simulink model "joint_impedance_control"  (R2019a)
settings: Solver=FixedStepDiscrete  StartTime=0.0  StopTime=inf  FixedStep=0.001  RelTol=1e-3
PreLoadFcn:
  | set_param(gcs, 'RTWSystemTargetFile', 'franka_emika_panda.tlc');
  | 
  | demos_common_configs();
  | collision_behavior = ones(1,52)*100;
libraries: franka_simulink_library x6, simulink x1
settings Model: SimulationMode=external  ExtModeTrigDuration=10000  Creator=vasi_ko  LastModifiedBy=konstantinosvasios
settings DataIOCC: LimitDataPoints=on  SaveFormat=Array  ReturnWorkspaceOutputs=off
settings OptimizationCC: EnhancedBackFolding=on  OptimizeBlockOrder=speed  DifferentSizesBufferReuse=on  OptimizationCustomize=off
settings DebuggingCC: SolverPrmCheckMsg=warning  ParameterTunabilityLossMsg=error  SFUnexpectedBacktrackingDiag=warning  SFNoUnconditionalDefaultTransitionDiag=warning  SFExecutionAtInitializationDiag=none  ArithmeticOperatorsInVariantConditions=warning
settings HardwareCC: ProdBitPerLong=64  ProdHWDeviceType=Intel->x86-64 (Linux 64)
settings ModelReferenceCC: PropagateSignalLabelsOutOfModel=off
settings SFSimCC: SimUseLocalCustomCode=off  MATLABDynamicMemAlloc=off
settings RTWCC: Description=Generic Real-Time Target  SystemTargetFile=franka_emika_panda.tlc  RTWUseLocalCustomCode=off  Toolchain=Franka Simulink | gmake (64-bit linux)  BuildConfiguration=Faster Runs  TargetLang=C++
settings CodeAppCC: OperatorAnnotations=on
settings STFCustomTargetCC: TargetLangStandard=C99 (ISO)  ModelReferenceCompliant=off  MatFileLogging=on  UseToolchainInfoCompliant=on  SystemTargetFile=franka_emika_panda.tlc
settings GRTTargetCC: ModelReferenceCompliant=off  ParMdlRefBuildCompliant=off  CompOptLevelCompliant=off  ConcurrentExecutionCompliant=off  CombineOutputUpdateFcns=off  CPPClassGenCompliant=off  GRTInterface=on  ExtModeTransport=1
settings ConfigComp: CovMetricSettings=dw  CovSaveCumulativeToWorkspaceVar=on  CovSaveSingleToWorkspaceVar=on  CovExternalEMLEnable=off  CovSFcnEnable=off

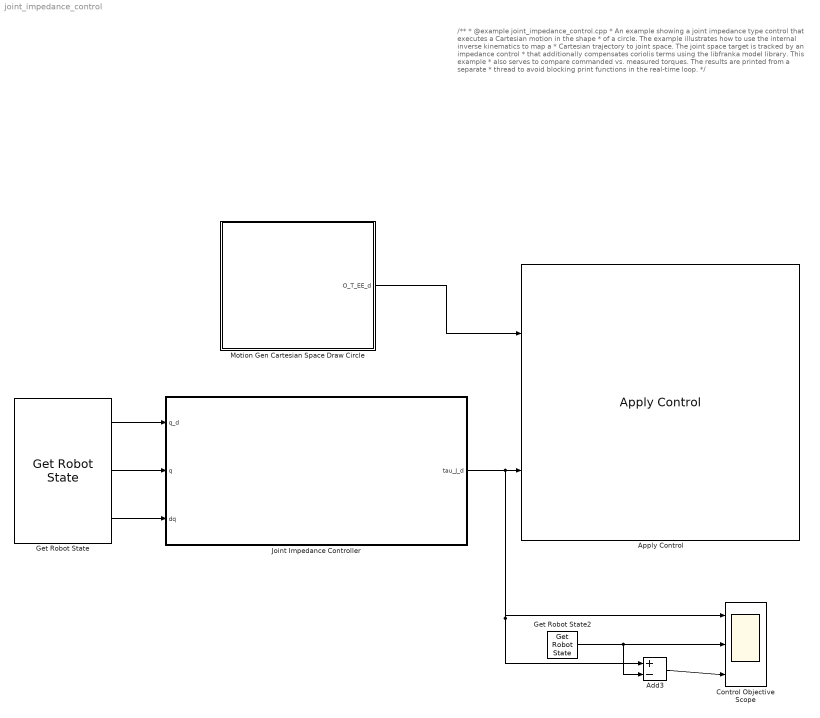
== system joint_impedance_control ==
  note: /**
      |  * @example joint_impedance_control.cpp
      |  * An example showing a joint impedance type control that executes a Cartesian motion in the shape
      |  * of a circle. The example illustrates how to use the internal inverse kinematics to map a
      |  * Cartesian trajectory to joint space. The joint space target is tracked by an impedance control
      |  * that additionally compensates coriolis terms using the libfranka model library. This example
      |  * also serves to compare commanded vs. measured torques. The results are printed from a separate
      |  * thread to avoid blocking print functions in the real-time loop.
      |  */
  Add3 : Sum  Inputs=+-
  Apply Control : franka_simulink_library/Apply Control  robot_ip=robot_ip  gripper_attached=off  control_mode=Torque Control - Cartesian Pose  controller_choice=Joint Impedance Controller  elbow_control=off  collision_thresholds=100*ones(1,52)  joint_impedance=joint_impedance  cartesian_impedance=cartesian_impedance  load_inertia=load_inertia  EE_T_K=EE_T_K  init_joint_configuration_req=on  init_joint_configuration=[0, -pi/4, 0, -3 * pi/4, 0, pi/2, pi/4]
      settings: SourceProductName=Franka Emika
  Control Objective Scope : Scope  NumInputPorts=3
  Get Robot State : franka_simulink_library/Get Robot State  robot_ip=robot_ip  signals_requested='q_d q dq'
      settings: SourceProductName=Franka Emika
  Get Robot State2 : franka_simulink_library/Get Robot State  robot_ip=robot_ip  signals_requested='tau_J'
      settings: SourceProductName=Franka Emika
  Joint Impedance Controller : Subsystem
      mask Display:
      | disp('{\bf\fontsize{18}Joint Impedance Controller}', 'texmode','on');
      | 
      | block_icon('Controller')
      | 
      | port_label('output',1,'tau_J_d');
      | 
      | port_label('input',1,'q_d');
      | port_label('input',2,'q');
      | port_label('input',3,'dq');
  Motion Gen Cartesian Space Draw Circle : Subsystem
      mask Display:
      | pos = get_param(gcb, 'Position');
      | width = pos(3) - pos(1);
      | x = [0:width];
      | y = sin(x/180*pi);
      | % Parameters 'm' and 'b' must be defined in 'Parameters & Dialog' pane.
      | plot((1/2)*cos(x/180*2*pi+pi/4), (1/2)*sin(x/180*2*pi+pi/4));
      | 
      | port_label('output',1,'O_T_EE_d');
  wires:
  Motion Gen Cartesian Space Draw Circle/1(O_T_EE_d) -> Apply Control/1
  Joint Impedance Controller/1(tau_J_d) -> Control Objective Scope/1, Add3/1, Apply Control/2
  Get Robot State/1 -> Joint Impedance Controller/1(q_d)
  Get Robot State/2 -> Joint Impedance Controller/2(q)
  Get Robot State/3 -> Joint Impedance Controller/3(dq)
  Get Robot State2/1 -> Add3/2, Control Objective Scope/2
  Add3/1 -> Control Objective Scope/3

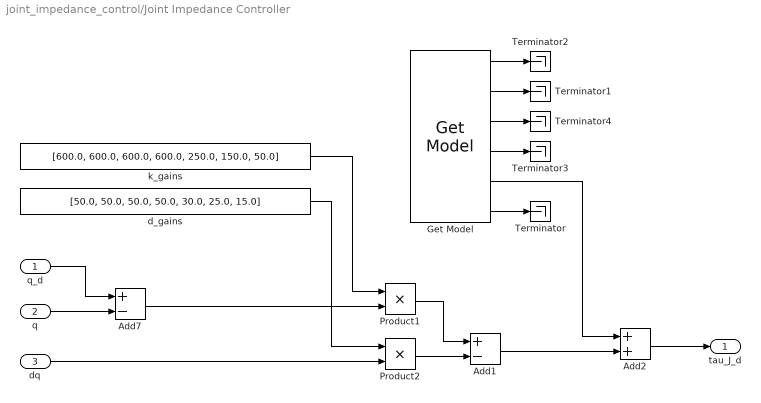
== system joint_impedance_control/Joint Impedance Controller ==
  q_d : Inport
  q : Inport  Port=2
  dq : Inport  Port=3
  Add1 : Sum  Inputs=+-
  Add2 : Sum
  Add7 : Sum  Inputs=+-
  Get Model : franka_simulink_library/Get Model  robot_ip=robot_ip
      settings: SourceProductName=Franka Emika Simulink Support Package
  Product1 : Product
  Product2 : Product
  Terminator{,1..4} (5 alike) : Terminator
  d_gains : Constant  Value=[50.0, 50.0, 50.0, 50.0, 30.0, 25.0, 15.0]  VectorParams1D=off
  k_gains : Constant  Value=[600.0, 600.0, 600.0, 600.0, 250.0, 150.0, 50.0]  VectorParams1D=off
  tau_J_d : Outport  VectorParamsAs1DForOutWhenUnconnected=off
  wires:
  Get Model/1 -> Terminator2/1
  Get Model/6 -> Terminator/1
  Get Model/4 -> Terminator3/1
  Get Model/2 -> Terminator1/1
  Get Model/3 -> Terminator4/1
  q_d/1 -> Add7/1
  q/1 -> Add7/2
  k_gains/1 -> Product1/1
  Add7/1 -> Product1/2
  Product1/1 -> Add1/1
  d_gains/1 -> Product2/1
  dq/1 -> Product2/2
  Product2/1 -> Add1/2
  Add2/1 -> tau_J_d/1
  Get Model/5 -> Add2/1
  Add1/1 -> Add2/2

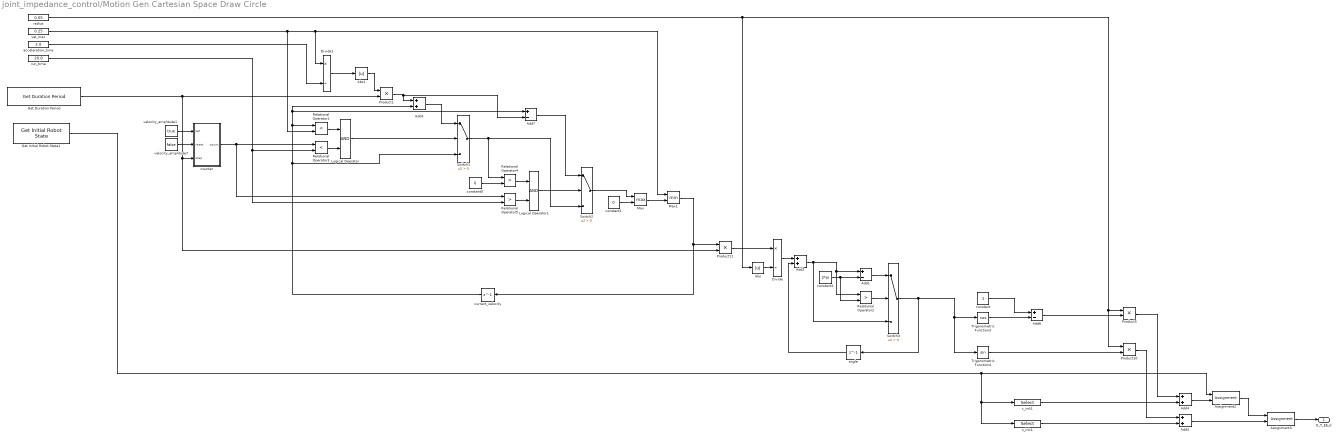
== system joint_impedance_control/Motion Gen Cartesian Space Draw Circle ==
  Abs : Abs
  Abs1 : Abs
  Add1 : Sum  Inputs=+-
  Add{2..5} (4 alike) : Sum
  Add6 : Sum  Inputs=+-
  Add7 : Sum  Inputs=+-
  Assignment2 : Assignment  DiagnosticForDimensions=Warning  IndexOptions=Index vector (dialog)  Indices=14  OutputSizes=1
  Assignment3 : Assignment  DiagnosticForDimensions=Warning  IndexOptions=Index vector (dialog)  Indices=15  OutputSizes=1
  Divide : Product  Inputs=*/
  Divide1 : Product  Inputs=*/
  Get Duration Period : franka_simulink_library/Get Duration Period  robot_ip=robot_ip
      settings: SourceProductName=Franka Emika
  Get Initial Robot State1 : franka_simulink_library/Get Initial Robot State  robot_ip=robot_ip  signals_requested='O_T_EE'
      settings: SourceProductName=Franka Emika
  Logical Operator : Logic  AllPortsSameDT=off  OutDataTypeStr=boolean
  Logical Operator1 : Logic  AllPortsSameDT=off  OutDataTypeStr=boolean
  Max : MinMax  Function=max  Inputs=2
  Max1 : MinMax  Inputs=2
  Product{1,5,10..11} (4 alike) : Product
  Relational Operator1 : RelationalOperator  Operator=<  OutDataTypeStr=boolean  RndMeth=Nearest
  Relational Operator2 : RelationalOperator  Operator=>  OutDataTypeStr=boolean  RndMeth=Nearest
  Relational Operator3 : RelationalOperator  Operator=<  OutDataTypeStr=boolean  RndMeth=Nearest
  Relational Operator4 : RelationalOperator  Operator=>  OutDataTypeStr=boolean  RndMeth=Nearest
  Relational Operator5 : RelationalOperator  Operator=>  OutDataTypeStr=boolean  RndMeth=Nearest
  Switch1 : Switch  Criteria=u2 > Threshold
  Switch2 : Switch  Criteria=u2 > Threshold
  Switch3 : Switch  Criteria=u2 > Threshold
  Trigonometric Function3 : Trigonometry  Operator=cos  NumberOfIterations=50
  Trigonometric Function4 : Trigonometry  NumberOfIterations=50
  acceleration_time : Constant  Value=2.0  VectorParams1D=off
  angle : Delay  DelayLength=1  InitialCondition=0
  constant : Constant  VectorParams1D=off
  constant0 : Constant  Value=0  VectorParams1D=off
  constant1 : Constant  Value=0  VectorParams1D=off
  constant2 : Constant  Value=2*pi  VectorParams1D=off
  counter : Subsystem
  current_velocity : Delay  DelayLength=1  InitialCondition=0
  radius : Constant  Value=0.05  VectorParams1D=off
  run_time : Constant  Value=20.0  VectorParams1D=off
  vel_max : Constant  Value=0.25  VectorParams1D=off
  velocity_amplitude1 : Constant  Value=true  VectorParams1D=off
  velocity_amplitude7 : Constant  Value=false  VectorParams1D=off
  x_init1 : Selector  InputPortWidth=16  IndexOptions=Index vector (dialog)  Indices=14  OutputSizes=1
  z_init1 : Selector  InputPortWidth=16  IndexOptions=Index vector (dialog)  Indices=15  OutputSizes=1
  O_T_EE_d : Outport  VectorParamsAs1DForOutWhenUnconnected=off
  wires:
  Get Duration Period/1 -> Product11/2, counter/3(step), Product1/2
  velocity_amplitude7/1 -> counter/2(reset)
  velocity_amplitude1/1 -> counter/1(set)
  x_init1/1 -> Add4/2
  Add5/1 -> Assignment3/2
  Get Initial Robot State1/1 -> z_init1/1, x_init1/1, Assignment2/1
  Product5/1 -> Add4/1
  z_init1/1 -> Add5/2
  Assignment3/1 -> O_T_EE_d/1
  Add4/1 -> Assignment2/2
  Assignment2/1 -> Assignment3/1
  radius/1 -> Product10/1, Product5/1, Abs/1
  Product10/1 -> Add5/1
  Trigonometric Function3/1 -> Add6/2
  constant/1 -> Add6/1
  Add6/1 -> Product5/2
  Trigonometric Function4/1 -> Product10/2
  vel_max/1 -> Max1/1, Divide1/1, Relational Operator1/2
  run_time/1 -> Relational Operator5/2, Relational Operator3/2
  counter/1(count) -> Relational Operator5/1, Relational Operator3/1
  Relational Operator3/1 -> Logical Operator/2
  Relational Operator1/1 -> Logical Operator/1
  Logical Operator/1 -> Switch1/2
  current_velocity/1 -> Switch1/3, Add7/1, Add3/2, Relational Operator1/1
  Logical Operator1/1 -> Switch2/2
  Switch1/1 -> Relational Operator4/1, Switch2/3
  Relational Operator5/1 -> Logical Operator1/2
  Relational Operator4/1 -> Logical Operator1/1
  constant0/1 -> Relational Operator4/2
  Switch2/1 -> Max/1
  constant1/1 -> Max/2
  Max/1 -> Max1/2
  Max1/1 -> current_velocity/1, Product11/1
  Abs/1 -> Divide/2
  Switch3/1 -> angle/1, Trigonometric Function4/1, Trigonometric Function3/1
  Add2/1 -> Relational Operator2/1, Add1/1, Switch3/3
  constant2/1 -> Relational Operator2/2, Add1/2
  Relational Operator2/1 -> Switch3/2
  Add1/1 -> Switch3/1
  Product11/1 -> Divide/1
  angle/1 -> Add2/2
  Divide1/1 -> Abs1/1
  acceleration_time/1 -> Divide1/2
  Abs1/1 -> Product1/1
  Product1/1 -> Add7/2, Add3/1
  Add3/1 -> Switch1/1
  Add7/1 -> Switch2/1
  Divide/1 -> Add2/1

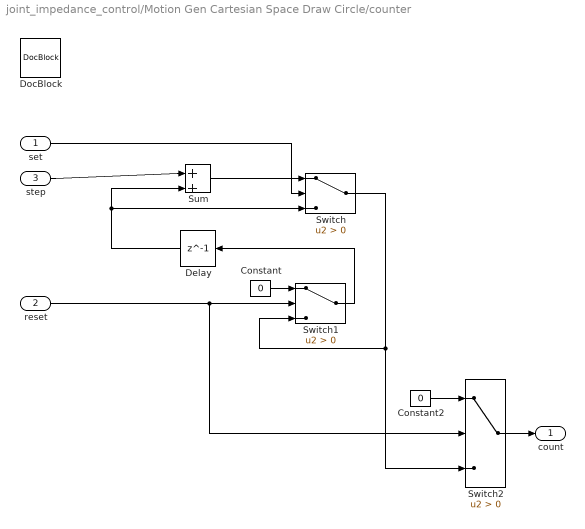
== system joint_impedance_control/Motion Gen Cartesian Space Draw Circle/counter ==
  set : Inport  OutDataTypeStr=boolean
  reset : Inport  Port=2  OutDataTypeStr=boolean
  step : Inport  Port=3  OutDataTypeStr=double
  Constant : Constant  Value=0  OutDataTypeStr=double
  Constant2 : Constant  Value=0  OutDataTypeStr=double
  Delay : Delay  DelayLength=1  InitialCondition=0
  DocBlock : simulink/Model-Wide Utilities/DocBlock  DocumentType=Text
      content=|
      | %% counter
      | %
      | % This library includes the counter functionality that increases
      | % it's output by an input step factor for each computational step. The counter
      | % can also be externaly reset.
      | % -----------------------------------------------------------------------
      | % Author    : Konstantinos Vasios
      | % Date      : 01.09.2017
      | % Copyright : Franka Emika GmbH
      | % -----------------------------------------------------------------------
      | %
      | % Inputs:
      | % @param set : activates the counter. (data type: boolean, dimension: 1)
      | % @param reset: it resets the counter. Count starts from 0. (data type: boolean, dimension: 1)
      | % @param step: increment factor. (data type: real, dimension: 1)
      | %
      | % Outputs:
      | % @return count: current counter value. (data type: real, dimension: 1)
      | %% -----------------------------------------------------------------------
  Sum : Sum  Inputs=|++
  Switch : Switch  Criteria=u2 > Threshold
  Switch1 : Switch  Criteria=u2 > Threshold  OutDataTypeStr=double
  Switch2 : Switch  Criteria=u2 > Threshold  OutDataTypeStr=double
  count : Outport  OutDataTypeStr=double  VectorParamsAs1DForOutWhenUnconnected=off
  wires:
  Switch1/1 -> Delay/1
  Constant/1 -> Switch1/1
  reset/1 -> Switch2/2, Switch1/2
  Delay/1 -> Switch/3, Sum/2
  step/1 -> Sum/1
  Switch/1 -> Switch2/3, Switch1/3
  set/1 -> Switch/2
  Sum/1 -> Switch/1
  Constant2/1 -> Switch2/1
  Switch2/1 -> count/1
